simulink model "RLC"  (R2013a)
settings: Solver=ode45  StartTime=0.0  StopTime=0.01  RelTol=1e-3
InitFcn:
  | R=536;
  | L=23.74e-3;
  | C=82.38e-9;
settings Model: Creator=LuisFernando  LastModifiedBy=LuisFernando

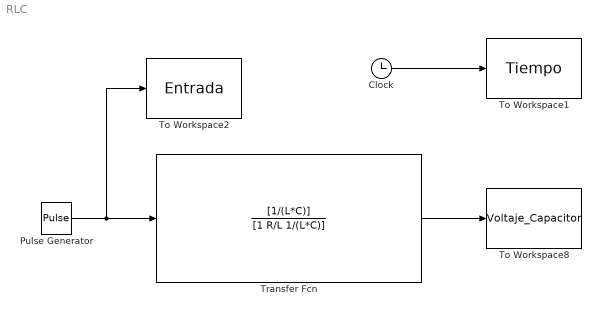
== system RLC ==
  Clock : Clock
      settings: Decimation=1000
  Pulse Generator : DiscretePulseGenerator  PulseType=Time based  Amplitude=5  Period=0.001360544  PulseWidth=5
  To Workspace1 : ToWorkspace  VariableName=Tiempo  SampleTime=-1
  To Workspace2 : ToWorkspace  VariableName=Entrada  SampleTime=-1
  To Workspace8 : ToWorkspace  VariableName=Voltaje_Capacitor  SampleTime=-1
  Transfer Fcn : TransferFcn  Numerator=[1/(L*C)]  Denominator=[1 R/L 1/(L*C)]
  wires:
  Transfer Fcn/1 -> To Workspace8/1
  Clock/1 -> To Workspace1/1
  Pulse Generator/1 -> To Workspace2/1, Transfer Fcn/1
